simulink model "SistemaAnalogicoCorrerelarchivoM"  (R2018a)
settings: Solver=VariableStepAuto  StartTime=0.0  StopTime=10.0  RelTol=1e-3
undefined symbols (not defined in the file or in its folder): dcgain, Gc, GiL, Gplanta, Hestim, integrador
settings Model: Creator=Ignacio  LastModifiedBy=Ignacio

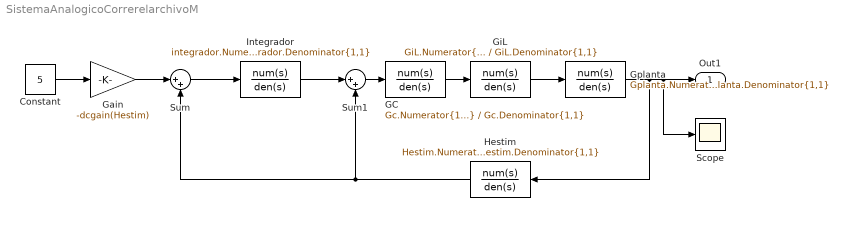
== system SistemaAnalogicoCorrerelarchivoM ==
  Constant : Constant  Value=5
  GC : TransferFcn  Numerator=Gc.Numerator{1,1}  Denominator=Gc.Denominator{1,1}
  Gain : Gain  Gain=-dcgain(Hestim)
  GiL : TransferFcn  Numerator=GiL.Numerator{1,1}  Denominator=GiL.Denominator{1,1}
  Gplanta : TransferFcn  Numerator=Gplanta.Numerator{1,1}  Denominator=Gplanta.Denominator{1,1}
  Hestim : TransferFcn  Numerator=Hestim.Numerator{1,1}  Denominator=Hestim.Denominator{1,1}
  Integrador : TransferFcn  Numerator=integrador.Numerator{1,1}  Denominator=integrador.Denominator{1,1}
  Scope : Scope
  Sum : Sum  Inputs=|++
  Sum1 : Sum  Inputs=|++
  Out1 : Outport
  wires:
  Constant/1 -> Gain/1
  Sum/1 -> Integrador/1
  Integrador/1 -> Sum1/1
  Sum1/1 -> GC/1
  GiL/1 -> Gplanta/1
  Hestim/1 -> Sum1/2, Sum/2
  Gplanta/1 -> Scope/1, Out1/1, Hestim/1
  GC/1 -> GiL/1
  Gain/1 -> Sum/1
